simulink model "airTrackLab"  (R2021a)
settings: Solver=ode23t  StartTime=0.0  StopTime=30  FixedStep=0.02  MaxStep=0.01  RelTol=1e-3  AbsTol=1e-4  EnableMultiTasking=on
PostLoadFcn:
  | disp('default settings')
  | 
  | % Default starting positions
  | x0_cart1 = -0.2
  | x0_cart2 = 0.8
  | x0_gate1 = -0.4
  | x0_gate2 = 0.4
  | 
  | % How much damping the carts feel
  | dampingCoef = 0.01 % N/(m/s)
  | 
  | % Hanger damping
  | pulleyDamping = 0;
  | 
  | % Max measurement noise for the gates
  | noise_max = 0.01 % seconds
  | 
  | % How many time steps to show in the history
  | nHistory = 4
  | 
  | % Based on the provided STLs
  | cart_length = 0.15
  | 
  | subsystems = find_system(gcs,'BlockType','SubSystem');
  | p = Simulink.Mask.get(subsystems{1});
  | p.Parameters(1).Value = '-0.8';
  | p.Parameters(2).Value = '0';
  | p.Parameters(3).Value = '-0.4';
  | p.Parameters(4).Value = '0.4';
  | p.Parameters(5).Value = '0';
  | p.Parameters(6).Value = '0';
  | 
  | % Resize the model window
  | set(0,"Units","pixels")
  | sSize = get(0,"screensize");
  | set_param(gcs,'location',...
  |     [1,sSize(4)*0.01,round(sSize(3)/2),sSize(4)*0.96]);
  | 
  | % Reset the zoom
  | set_param(gcs, 'ZoomFactor','FitSystem')
undefined symbols (not defined in the file): X, Y, Z
libraries: sm_lib x104, simulink x12, nesl_utility x9
(part 2 of 3)

== system airTrackLab/Air track model/Endstop R ==
  File Solid2 : sm_lib/Body Elements/File Solid  ExtGeomFileName=wheel_stop.stl  UnitType=Custom  ExtGeomFileUnits=mm  StepReaderType=HEX  ExportConvexHullGeometry=off  InertiaType=PointMass  Mass=180  MassUnits=g  CenterOfMass=[0 0 0]  CenterOfMassUnits=m  MomentsOfInertia=[1 1 1]  MomentsOfInertiaUnits=kg*m^2  ProductsOfInertia=[0 0 0]  ProductsOfInertiaUnits=kg*m^2  BasedOnType=Density  Density=1000  DensityUnits=kg/m^3  DoExposeReferenceFrame=on  SerializedFrames=<Frames><Frame><Id>Frame1</Id><Value><Name>F1</Name><Origin><Source>CenterOfMassFrame</Source><FeatureName></FeatureName></Origin><PrimaryAxis><DefinedDirection>+X</DefinedDirection><Source>ReferenceFrame</Source><SourceDirection>+Z</SourceDirection><FeatureName></FeatureName></PrimaryAxis><SecondaryAxis><DefinedDirection>+Y</DefinedDirection><Source>ReferenceFrame</Source><SourceDirection>+X</SourceDirection><FeatureName></FeatureName></SecondaryAxis></Value></Frame></Frames>  GraphicType=FromGeometry  MarkerShape=Sphere  MarkerSize=10  GraphicVisPropType=AdvancedVisualProperties  GraphicDiffuseColor="[0.2   0.2    0.2]"  GraphicSpecularColor="[0.8    0.8   0.8 1]"  GraphicAmbientColor=[0.05 0.05 0.05 1]  GraphicEmissiveColor=[0.0 0.0 0.0 1.0]  GraphicShininess=50  GraphicOpacity=1.0
  Rigid Transform1 : sm_lib/Frames and Transforms/Rigid Transform  TranslationMethod=Cartesian  TranslationStandardOffset=1  TranslationLengthUnit=m  TranslationStandardAxis=+X  TranslationCartesianOffset=[1-0.012 -0.225 0]  TranslationROffset=0  TranslationROffsetUnits=m  TranslationZOffset=0  TranslationZOffsetUnits=m  TranslationThetaOffset=0  TranslationThetaOffsetUnits=deg  RotationMethod=None  RotationAngleUnits=deg  RotationStandardAxis=+Z  RotationAngle=0.0  RotationArbitraryAxis=[0 0 1]  FollAlignAxisA=+X  BaseAlignAxisA=+Y  FollAlignAxisB=+Y  BaseAlignAxisB=+Z  RotationSequenceAxes=FollowerAxes  RotationSequence=XYX  RotationSequenceAngles=[0 0 0]  RotationSequenceAnglesUnits=deg  RotationMatrix=[1 0 0; 0 1 0; 0 0 1]
  contact_ball1 : sm_lib/Body Elements/Spherical Solid  GraphicAmbientColor=[0.15 0.15 0.15 1.0]  BasedOnType=Density  CenterOfMass=[0 0 0]  CenterOfMassUnits=m  GraphicDiffuseColor="[ 0.9290    0.6940    0.1250]"  Density=1000  DensityUnits=kg/m^3  DoExposeReferenceFrame=on  GraphicEmissiveColor=[0.0 0.0 0.0 1.0]  ExportEntireGeometry=on  SerializedExposedGeometries=<ExposedGeometries><ExposedGeometry><RawGeometryId>entire</RawGeometryId><ExposedGeometryId>G</ExposedGeometryId></ExposedGeometry></ExposedGeometries>  SerializedFrames=<Frames/>  MarkerShape=Sphere  MarkerSize=10  GraphicType=FromGeometry  InertiaType=CalculateFromGeometry  Mass=1  MassUnits=kg  MomentsOfInertia=[1 1 1]  MomentsOfInertiaUnits=kg*m^2  GraphicOpacity=1.0  ProductsOfInertia=[0 0 0]  ProductsOfInertiaUnits=kg*m^2  GraphicShininess=75  GraphicSpecularColor=[0.5 0.5 0.5 1.0]  SphereRadius=0.0075  SphereRadiusUnits=m  GraphicVisPropType=SimpleVisualProperties
  C : PMIOPort  Side=Left
  R : PMIOPort  Port=2  Side=Right
  connections:
  File Solid2/RConn1 -- C/RConn1 -- Rigid Transform1/RConn1 -- R/RConn1
  contact_ball1/RConn1 -- Rigid Transform1/LConn1

== system airTrackLab/Air track model/Force Cart 1 ==
  Add1 : Sum  Inputs=+++
  Force Factor : Gain  Gain=0.5
  Push+ : Constant  SampleTime=-1
  Push- : Constant  Value=-1  SampleTime=-1
  Simulink-PS Converter : nesl_utility/Simulink-PS Converter  PhysicalDomain=network_engine_domain  SubClassName=ps_input  LeftPortType=input  RightPortType=output  PseudoPeriodic=off  Frequencies=[]  NoiseDistribution=none  NoiseParameters=[]  Unit=1  AffineConversion=off  FilteringAndDerivatives=provide  SimscapeFilterOrder=1  InputFilterTimeConstant=0.001  UdotUserProvided=0
      settings: SourceProductBaseCode=PW,SS
  on1+ : Gain  Gain=0
  on1- : Gain  Gain=0
  short pulse : Subsystem
  f : PMIOPort  Side=Right
  wires:
  Force Factor/1 -> Simulink-PS Converter/1
  on1+/1 -> Add1/2
  Push-/1 -> on1-/1
  Push+/1 -> on1+/1
  on1-/1 -> Add1/1
  Add1/1 -> Force Factor/1
  short pulse/1(Out1) -> Add1/3
  connections:
  Simulink-PS Converter/RConn1 -- f/RConn1

== system airTrackLab/Air track model/Force Cart 2 ==
  Add : Sum  Inputs=+++
  Force Factor C2 : Gain  Gain=0.5
  Interactive Pulse : Subsystem
  Push+ : Constant  SampleTime=-1
  Push- : Constant  Value=-1  SampleTime=-1
  Simulink-PS Converter1 : nesl_utility/Simulink-PS Converter  PhysicalDomain=network_engine_domain  SubClassName=ps_input  LeftPortType=input  RightPortType=output  PseudoPeriodic=off  Frequencies=[]  NoiseDistribution=none  NoiseParameters=[]  Unit=1  AffineConversion=off  FilteringAndDerivatives=provide  SimscapeFilterOrder=1  InputFilterTimeConstant=0.001  UdotUserProvided=0
      settings: SourceProductBaseCode=PW,SS
  on2+ : Gain  Gain=0
  on2- : Gain  Gain=0
  f : PMIOPort  Side=Right
  wires:
  Add/1 -> Force Factor C2/1
  Interactive Pulse/1(Out1) -> Add/3
  Force Factor C2/1 -> Simulink-PS Converter1/1
  Push+/1 -> on2+/1
  Push-/1 -> on2-/1
  on2-/1 -> Add/1
  on2+/1 -> Add/2
  connections:
  f/RConn1 -- Simulink-PS Converter1/RConn1

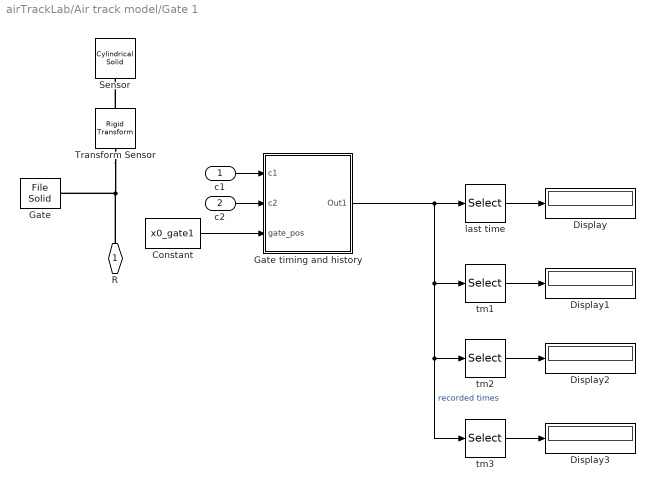
== system airTrackLab/Air track model/Gate 1 ==
  c1 : Inport
  c2 : Inport  Port=2
  Constant : Constant  Value=x0_gate1
  Display{,1..3} (4 alike) : Display
  Gate : sm_lib/Body Elements/File Solid  ExtGeomFileName=gate.stl  UnitType=Custom  ExtGeomFileUnits=mm  StepReaderType=HEX  ExportConvexHullGeometry=off  InertiaType=PointMass  Mass=180  MassUnits=g  CenterOfMass=[0 0 0]  CenterOfMassUnits=m  MomentsOfInertia=[1 1 1]  MomentsOfInertiaUnits=kg*m^2  ProductsOfInertia=[0 0 0]  ProductsOfInertiaUnits=kg*m^2  BasedOnType=Density  Density=1000  DensityUnits=kg/m^3  DoExposeReferenceFrame=on  SerializedFrames=<Frames/>  GraphicType=FromGeometry  MarkerShape=Sphere  MarkerSize=10  GraphicVisPropType=SimpleVisualProperties  GraphicDiffuseColor="[0.8500    0.3250    0.0980]"  GraphicSpecularColor="[0.8    0.8   0.8 1]"  GraphicAmbientColor=[0.05 0.05 0.05 1]  GraphicEmissiveColor=[0.0 0.0 0.0 1.0]  GraphicShininess=50  GraphicOpacity=0.5
  Gate timing and history : Subsystem
  Sensor : sm_lib/Body Elements/Cylindrical Solid  GraphicAmbientColor=[0.15 0.15 0.15 1.0]  BasedOnType=Density  CenterOfMass=[0 0 0]  CenterOfMassUnits=m  GraphicDiffuseColor=[0.0 0.6 0.0]  CylinderLength=0.008  CylinderLengthUnits=m  CylinderRadius=0.01  CylinderRadiusUnits=m  Density=1000  DensityUnits=kg/m^3  DoExposeReferenceFrame=on  GraphicEmissiveColor=[0.0 0.0 0.0 1.0]  ExportEntireGeometry=off  SerializedFrames=<Frames/>  MarkerShape=Sphere  MarkerSize=10  GraphicType=FromGeometry  InertiaType=CalculateFromGeometry  Mass=1  MassUnits=kg  MomentsOfInertia=[1 1 1]  MomentsOfInertiaUnits=kg*m^2  GraphicOpacity=1.0  ProductsOfInertia=[0 0 0]  ProductsOfInertiaUnits=kg*m^2  GraphicShininess=75  GraphicSpecularColor=[0.5 0.5 0.5 1.0]  GraphicVisPropType=SimpleVisualProperties
  Transform Sensor : sm_lib/Frames and Transforms/Rigid Transform  TranslationMethod=StandardAxis  TranslationStandardOffset=0.2675  TranslationLengthUnit=m  TranslationStandardAxis=+Y  TranslationCartesianOffset=[0 0 0]  TranslationROffset=0  TranslationROffsetUnits=m  TranslationZOffset=0  TranslationZOffsetUnits=m  TranslationThetaOffset=0  TranslationThetaOffsetUnits=deg  RotationMethod=StandardAxis  RotationAngleUnits=deg  RotationStandardAxis=+X  RotationAngle=-90  RotationArbitraryAxis=[0 0 1]  FollAlignAxisA=+X  BaseAlignAxisA=+Y  FollAlignAxisB=+Y  BaseAlignAxisB=+Z  RotationSequenceAxes=FollowerAxes  RotationSequence=XYX  RotationSequenceAngles=[0 0 0]  RotationSequenceAnglesUnits=deg  RotationMatrix=[1 0 0; 0 1 0; 0 0 1]
  last time : Selector  InputPortWidth=4  IndexOptions=Index vector (dialog)  Indices=1  OutputSizes=1
  tm1 : Selector  InputPortWidth=4  IndexOptions=Index vector (dialog)  Indices=2  OutputSizes=1
  tm2 : Selector  InputPortWidth=4  IndexOptions=Index vector (dialog)  Indices=3  OutputSizes=1
  tm3 : Selector  InputPortWidth=4  IndexOptions=Index vector (dialog)  Indices=4  OutputSizes=1
  R : PMIOPort  Side=Right
  wires:
  Gate timing and history/1(Out1) -> tm3/1, tm2/1, tm1/1, last time/1  "recorded times"
  Constant/1 -> Gate timing and history/3(gate_pos)
  c1/1 -> Gate timing and history/1(c1)
  c2/1 -> Gate timing and history/2(c2)
  last time/1 -> Display/1
  tm1/1 -> Display1/1
  tm2/1 -> Display2/1
  tm3/1 -> Display3/1
  connections:
  R/RConn1 -- Transform Sensor/LConn1 -- Gate/RConn1
  Transform Sensor/RConn1 -- Sensor/RConn1

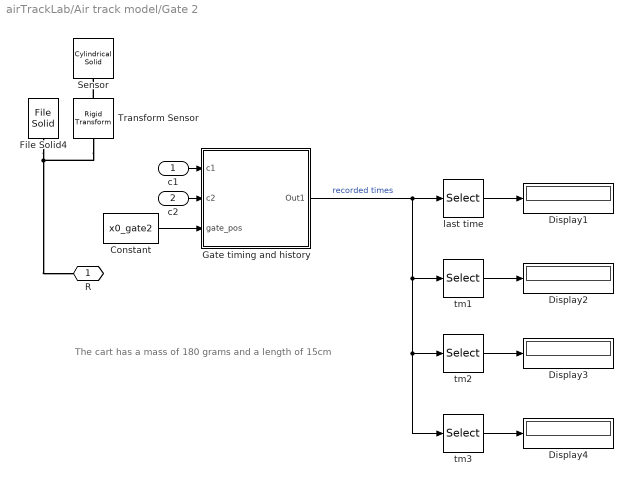
== system airTrackLab/Air track model/Gate 2 ==
  note: The cart has a mass of 180 grams and a length of 15cm
  c1 : Inport
  c2 : Inport  Port=2
  Constant : Constant  Value=x0_gate2
  Display{1..4} (4 alike) : Display
  File Solid4 : sm_lib/Body Elements/File Solid  ExtGeomFileName=gate.stl  UnitType=Custom  ExtGeomFileUnits=mm  StepReaderType=HEX  ExportConvexHullGeometry=off  InertiaType=PointMass  Mass=180  MassUnits=g  CenterOfMass=[0 0 0]  CenterOfMassUnits=m  MomentsOfInertia=[1 1 1]  MomentsOfInertiaUnits=kg*m^2  ProductsOfInertia=[0 0 0]  ProductsOfInertiaUnits=kg*m^2  BasedOnType=Density  Density=1000  DensityUnits=kg/m^3  DoExposeReferenceFrame=on  SerializedFrames=<Frames/>  GraphicType=FromGeometry  MarkerShape=Sphere  MarkerSize=10  GraphicVisPropType=SimpleVisualProperties  GraphicDiffuseColor="[           0    0.4470    0.7410]"  GraphicSpecularColor="[0.8    0.8   0.8 1]"  GraphicAmbientColor=[0.05 0.05 0.05 1]  GraphicEmissiveColor=[0.0 0.0 0.0 1.0]  GraphicShininess=50  GraphicOpacity=0.5
  Gate timing and history : Subsystem
  Sensor : sm_lib/Body Elements/Cylindrical Solid  GraphicAmbientColor=[0.15 0.15 0.15 1.0]  BasedOnType=Density  CenterOfMass=[0 0 0]  CenterOfMassUnits=m  GraphicDiffuseColor=[0.0 0.6 0.0]  CylinderLength=0.008  CylinderLengthUnits=m  CylinderRadius=0.01  CylinderRadiusUnits=m  Density=1000  DensityUnits=kg/m^3  DoExposeReferenceFrame=on  GraphicEmissiveColor=[0.0 0.0 0.0 1.0]  ExportEntireGeometry=off  SerializedFrames=<Frames/>  MarkerShape=Sphere  MarkerSize=10  GraphicType=FromGeometry  InertiaType=CalculateFromGeometry  Mass=1  MassUnits=kg  MomentsOfInertia=[1 1 1]  MomentsOfInertiaUnits=kg*m^2  GraphicOpacity=1.0  ProductsOfInertia=[0 0 0]  ProductsOfInertiaUnits=kg*m^2  GraphicShininess=75  GraphicSpecularColor=[0.5 0.5 0.5 1.0]  GraphicVisPropType=SimpleVisualProperties
  Transform Sensor : sm_lib/Frames and Transforms/Rigid Transform  TranslationMethod=StandardAxis  TranslationStandardOffset=0.2675  TranslationLengthUnit=m  TranslationStandardAxis=+Y  TranslationCartesianOffset=[0 0 0]  TranslationROffset=0  TranslationROffsetUnits=m  TranslationZOffset=0  TranslationZOffsetUnits=m  TranslationThetaOffset=0  TranslationThetaOffsetUnits=deg  RotationMethod=StandardAxis  RotationAngleUnits=deg  RotationStandardAxis=+X  RotationAngle=-90  RotationArbitraryAxis=[0 0 1]  FollAlignAxisA=+X  BaseAlignAxisA=+Y  FollAlignAxisB=+Y  BaseAlignAxisB=+Z  RotationSequenceAxes=FollowerAxes  RotationSequence=XYX  RotationSequenceAngles=[0 0 0]  RotationSequenceAnglesUnits=deg  RotationMatrix=[1 0 0; 0 1 0; 0 0 1]
  last time : Selector  InputPortWidth=4  IndexOptions=Index vector (dialog)  Indices=1  OutputSizes=1
  tm1 : Selector  InputPortWidth=4  IndexOptions=Index vector (dialog)  Indices=2  OutputSizes=1
  tm2 : Selector  InputPortWidth=4  IndexOptions=Index vector (dialog)  Indices=3  OutputSizes=1
  tm3 : Selector  InputPortWidth=4  IndexOptions=Index vector (dialog)  Indices=4  OutputSizes=1
  R : PMIOPort  Side=Right
  wires:
  Constant/1 -> Gate timing and history/3(gate_pos)
  c1/1 -> Gate timing and history/1(c1)
  c2/1 -> Gate timing and history/2(c2)
  Gate timing and history/1(Out1) -> tm3/1, tm2/1, tm1/1, last time/1  "recorded times"
  tm1/1 -> Display2/1
  tm3/1 -> Display4/1
  last time/1 -> Display1/1
  tm2/1 -> Display3/1
  connections:
  File Solid4/RConn1 -- Transform Sensor/LConn1 -- R/RConn1
  Transform Sensor/RConn1 -- Sensor/RConn1

== system airTrackLab/Air track model/Load ==
  Hanging Mass : Subsystem  VariantControl=Hanging_Mass
  None : Subsystem  VariantControl=None
  Cable : PMIOPort  Side=Left
  Bracket : PMIOPort  Port=2  Side=Left

== system airTrackLab/Air track model/Mass Cart 1 ==
  "None " : Subsystem  VariantControl=None
      mask Display: disp(' ');
  Plates 1 : Subsystem  VariantControl=Plates_1
      mask Display: image('Plates_1.png');
  Plates 2 : Subsystem  VariantControl=Plates_2
      mask Display: image('Plates_2.png');
  Plates 3 : Subsystem  VariantControl=Plates_3
      mask Display: image('Plates_3.png');
  B : PMIOPort  Side=Right

== system airTrackLab/Air track model/Mass Cart 2 ==
  "None " : Subsystem  VariantControl=None
      mask Display: disp(' ');
  Plates 1 : Subsystem  VariantControl=Plates_1
      mask Display: image('Plates_1.png');
  Plates 2 : Subsystem  VariantControl=Plates_2
      mask Display: image('Plates_2.png');
  Plates 3 : Subsystem  VariantControl=Plates_3
      mask Display: image('Plates_3.png');
  B : PMIOPort  Side=Right

== system airTrackLab/Air track model/Subsystem1 ==
  Bus Creator : BusCreator  Inputs=2
  PS-Simulink Converter : nesl_utility/PS-Simulink Converter  PhysicalDomain=network_engine_domain  SubClassName=ps_output  LeftPortType=input  RightPortType=output  PseudoPeriodic=off  Frequencies=[]  Unit=inherit  AffineConversion=off
      settings: SourceProductBaseCode=PW,SS
  PS-Simulink Converter1 : nesl_utility/PS-Simulink Converter  PhysicalDomain=network_engine_domain  SubClassName=ps_output  LeftPortType=input  RightPortType=output  PseudoPeriodic=off  Frequencies=[]  Unit=inherit  AffineConversion=off
      settings: SourceProductBaseCode=PW,SS
  p : PMIOPort  Side=Left
  v : PMIOPort  Port=2  Side=Left
  pv : Outport
  wires:
  PS-Simulink Converter1/1 -> Bus Creator/1  "p"
  PS-Simulink Converter/1 -> Bus Creator/2  "v"
  Bus Creator/1 -> pv/1  "cart1"
  connections:
  v/RConn1 -- PS-Simulink Converter/LConn1
  p/RConn1 -- PS-Simulink Converter1/LConn1

== system airTrackLab/Air track model/Subsystem4 ==
  Bus Creator : BusCreator  Inputs=2
  PS-Simulink Converter : nesl_utility/PS-Simulink Converter  PhysicalDomain=network_engine_domain  SubClassName=ps_output  LeftPortType=input  RightPortType=output  PseudoPeriodic=off  Frequencies=[]  Unit=inherit  AffineConversion=off
      settings: SourceProductBaseCode=PW,SS
  PS-Simulink Converter1 : nesl_utility/PS-Simulink Converter  PhysicalDomain=network_engine_domain  SubClassName=ps_output  LeftPortType=input  RightPortType=output  PseudoPeriodic=off  Frequencies=[]  Unit=inherit  AffineConversion=off
      settings: SourceProductBaseCode=PW,SS
  p : PMIOPort  Side=Left
  v : PMIOPort  Port=2  Side=Left
  pv : Outport
  wires:
  Bus Creator/1 -> pv/1  "cart2"
  PS-Simulink Converter/1 -> Bus Creator/2  "v"
  PS-Simulink Converter1/1 -> Bus Creator/1  "p"
  connections:
  PS-Simulink Converter/LConn1 -- v/RConn1
  PS-Simulink Converter1/LConn1 -- p/RConn1

== system airTrackLab/Air track model/Contact Force/Elastic ==
  Contact Force Carts : sm_lib/Forces and Torques/Spatial Contact Force  CoefficientOfDynamicFriction=0.3  CoefficientOfStaticFriction=0.5  SenseContactBaseRotation=off  SenseContactBaseTranslation=off  NormalDamping=1e-3  NormalDampingUnits=N/(m/s)  SenseContactFollowerRotation=off  SenseContactFollowerTranslation=off  SenseContactSignal=off  NormalStiffness=1e9  NormalStiffnessUnits=N/m  FrictionalCriticalVelocity=1e-3  FrictionalCriticalVelocityUnits=m/s  ZeroCrossDetectContactStartAndEnd=off  FrictionType=None  SenseFrictionalForceMagnitude=off  SenseNormalForceMagnitude=off  NormalForceType=SmoothSpringDamper  SenseNormalVelocity=off  SenseSeparationDistance=off  SenseTangentialVelocity=off  SenseTangentialVelocityMagnitude=off  NormalTransitionRegionWidth=1e-4  NormalTransitionRegionWidthUnits=m
  Contact Force Carts1 : sm_lib/Forces and Torques/Spatial Contact Force  CoefficientOfDynamicFriction=0.3  CoefficientOfStaticFriction=0.5  SenseContactBaseRotation=off  SenseContactBaseTranslation=off  NormalDamping=1e-3  NormalDampingUnits=N/(m/s)  SenseContactFollowerRotation=off  SenseContactFollowerTranslation=off  SenseContactSignal=off  NormalStiffness=1e9  NormalStiffnessUnits=N/m  FrictionalCriticalVelocity=1e-3  FrictionalCriticalVelocityUnits=m/s  ZeroCrossDetectContactStartAndEnd=off  FrictionType=None  SenseFrictionalForceMagnitude=off  SenseNormalForceMagnitude=off  NormalForceType=SmoothSpringDamper  SenseNormalVelocity=off  SenseSeparationDistance=off  SenseTangentialVelocity=off  SenseTangentialVelocityMagnitude=off  NormalTransitionRegionWidth=1e-4  NormalTransitionRegionWidthUnits=m
  Reference Frame : sm_lib/Frames and Transforms/Reference Frame
  Reference Frame1 : sm_lib/Frames and Transforms/Reference Frame
  Weld Joint : sm_lib/Joints/Weld Joint  JointMode=ProvidedByInput  SenseConstraintForce=off  SenseConstraintForceX=off  SenseConstraintForceY=off  SenseConstraintForceZ=off  SenseConstraintTorque=off  SenseConstraintTorqueX=off  SenseConstraintTorqueY=off  SenseConstraintTorqueZ=off  SenseTotalForce=off  SenseTotalForceX=off  SenseTotalForceY=off  SenseTotalForceZ=off  SenseTotalTorque=off  SenseTotalTorqueX=off  SenseTotalTorqueY=off  SenseTotalTorqueZ=off  CompositeWrenchDir=FollowerOnBase  CompositeWrenchFrame=BaseFrame
  G1 : PMIOPort  Side=Left
  G2 : PMIOPort  Port=2  Side=Right
  F1 : PMIOPort  Port=3  Side=Left
  F2 : PMIOPort  Port=4  Side=Right
  connections:
  F1/RConn1 -- Reference Frame/RConn1
  F2/RConn1 -- Reference Frame1/RConn1
  G1/RConn1 -- Contact Force Carts/RConn1
  G2/RConn1 -- Contact Force Carts/LConn1

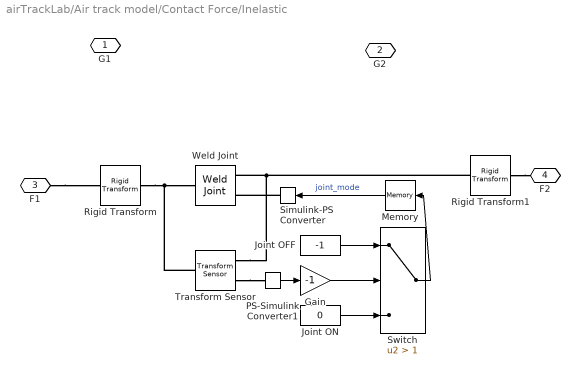
== system airTrackLab/Air track model/Contact Force/Inelastic ==
  Gain : Gain  Gain=-1
  Joint OFF : Constant  Value=-1
  Joint ON : Constant  Value=0
  Memory : Memory  InitialCondition=-1
  PS-Simulink Converter1 : nesl_utility/PS-Simulink Converter  PhysicalDomain=network_engine_domain  SubClassName=ps_output  LeftPortType=input  RightPortType=output  PseudoPeriodic=off  Frequencies=[]  Unit=mm  AffineConversion=off
      settings: SourceProductBaseCode=PW,SS
  Rigid Transform : sm_lib/Frames and Transforms/Rigid Transform  TranslationMethod=StandardAxis  TranslationStandardOffset=-0.075-0.0075  TranslationLengthUnit=m  TranslationStandardAxis=+Z  TranslationCartesianOffset=[0 0 0]  TranslationROffset=0  TranslationROffsetUnits=m  TranslationZOffset=0  TranslationZOffsetUnits=m  TranslationThetaOffset=0  TranslationThetaOffsetUnits=deg  RotationMethod=None  RotationAngleUnits=deg  RotationStandardAxis=+Z  RotationAngle=0.0  RotationArbitraryAxis=[0 0 1]  FollAlignAxisA=+X  BaseAlignAxisA=+Y  FollAlignAxisB=+Y  BaseAlignAxisB=+Z  RotationSequenceAxes=FollowerAxes  RotationSequence=XYX  RotationSequenceAngles=[0 0 0]  RotationSequenceAnglesUnits=deg  RotationMatrix=[1 0 0; 0 1 0; 0 0 1]
  Rigid Transform1 : sm_lib/Frames and Transforms/Rigid Transform  TranslationMethod=StandardAxis  TranslationStandardOffset=0.075+0.0075  TranslationLengthUnit=m  TranslationStandardAxis=+Z  TranslationCartesianOffset=[0 0 0]  TranslationROffset=0  TranslationROffsetUnits=m  TranslationZOffset=0  TranslationZOffsetUnits=m  TranslationThetaOffset=0  TranslationThetaOffsetUnits=deg  RotationMethod=None  RotationAngleUnits=deg  RotationStandardAxis=+Z  RotationAngle=0.0  RotationArbitraryAxis=[0 0 1]  FollAlignAxisA=+X  BaseAlignAxisA=+Y  FollAlignAxisB=+Y  BaseAlignAxisB=+Z  RotationSequenceAxes=FollowerAxes  RotationSequence=XYX  RotationSequenceAngles=[0 0 0]  RotationSequenceAnglesUnits=deg  RotationMatrix=[1 0 0; 0 1 0; 0 0 1]
  Simulink-PS Converter : nesl_utility/Simulink-PS Converter  PhysicalDomain=network_engine_domain  SubClassName=ps_input  LeftPortType=input  RightPortType=output  PseudoPeriodic=off  Frequencies=[]  NoiseDistribution=none  NoiseParameters=[]  Unit=1  AffineConversion=off  FilteringAndDerivatives=provide  SimscapeFilterOrder=1  InputFilterTimeConstant=0.001  UdotUserProvided=0
      settings: SourceProductBaseCode=PW,SS
  Switch : Switch  Criteria=u2 > Threshold  Threshold=1
  Transform Sensor : sm_lib/Frames and Transforms/Transform Sensor  MeasurementFrame=Base  SenseAngle=off  SenseAxis=off  SenseAngle1=off  SenseAngle2=off  SenseAngle3=off  SenseQ=off  SenseR=off  SenseOmegaX=off  SenseOmegaY=off  SenseOmegaZ=off  SenseOmega1=off  SenseOmega2=off  SenseOmega3=off  SenseQDot=off  SenseRDot=off  SenseAlphaX=off  SenseAlphaY=off  SenseAlphaZ=off  SenseAlpha1=off  SenseAlpha2=off  SenseAlpha3=off  SenseQDDot=off  SenseRDDot=off  SenseX=off  SenseY=off  SenseZ=on  SenseRad=off  SenseAzim=off  SenseDist=off  SenseInc=off  SenseXDot=off  SenseYDot=off  SenseZDot=off  SenseRadDot=off  SenseAzimDot=off  SenseDistDot=off  SenseIncDot=off  SenseXDDot=off  SenseYDDot=off  SenseZDDot=off  SenseRadDDot=off  SenseAzimDDot=off  SenseDistDDot=off  SenseIncDDot=off
  Weld Joint : sm_lib/Joints/Weld Joint  JointMode=ProvidedByInput  SenseConstraintForce=off  SenseConstraintForceX=off  SenseConstraintForceY=off  SenseConstraintForceZ=off  SenseConstraintTorque=off  SenseConstraintTorqueX=off  SenseConstraintTorqueY=off  SenseConstraintTorqueZ=off  SenseTotalForce=off  SenseTotalForceX=off  SenseTotalForceY=off  SenseTotalForceZ=off  SenseTotalTorque=off  SenseTotalTorqueX=off  SenseTotalTorqueY=off  SenseTotalTorqueZ=off  CompositeWrenchDir=FollowerOnBase  CompositeWrenchFrame=BaseFrame
  G1 : PMIOPort  Side=Left
  G2 : PMIOPort  Port=2  Side=Right
  F1 : PMIOPort  Port=3  Side=Left
  F2 : PMIOPort  Port=4  Side=Right
  wires:
  Joint OFF/1 -> Switch/1
  Joint ON/1 -> Switch/3
  Memory/1 -> Simulink-PS Converter/1  "joint_mode"
  Switch/1 -> Memory/1
  PS-Simulink Converter1/1 -> Gain/1
  Gain/1 -> Switch/2
  connections:
  Rigid Transform1/LConn1 -- F2/RConn1
  Simulink-PS Converter/RConn1 -- Weld Joint/LConn2
  F1/RConn1 -- Rigid Transform/LConn1
  Rigid Transform/RConn1 -- Transform Sensor/LConn1 -- Weld Joint/RConn1
  Rigid Transform1/RConn1 -- Transform Sensor/RConn1 -- Weld Joint/LConn1
  Transform Sensor/RConn2 -- PS-Simulink Converter1/LConn1

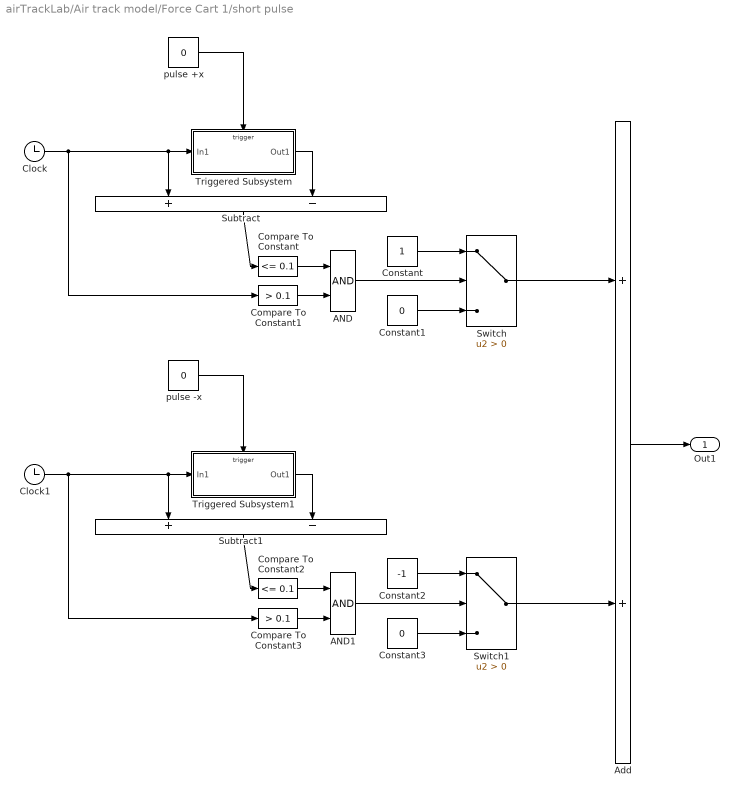
== system airTrackLab/Air track model/Force Cart 1/short pulse ==
  AND : Logic  IconShape=distinctive  AllPortsSameDT=off  OutDataTypeStr=boolean
  AND1 : Logic  IconShape=distinctive  AllPortsSameDT=off  OutDataTypeStr=boolean
  Add : Sum
  Clock : Clock
  Clock1 : Clock
  Compare To Constant : simulink/Logic and Bit Operations/Compare To Constant  relop=<=  const=0.1  OutDataTypeStr=boolean
  Compare To Constant1 : simulink/Logic and Bit Operations/Compare To Constant  relop=>  const=0.1  OutDataTypeStr=boolean
  Compare To Constant2 : simulink/Logic and Bit Operations/Compare To Constant  relop=<=  const=0.1  OutDataTypeStr=boolean
  Compare To Constant3 : simulink/Logic and Bit Operations/Compare To Constant  relop=>  const=0.1  OutDataTypeStr=boolean
  Constant : Constant
  Constant1 : Constant  Value=0
  Constant2 : Constant  Value=-1
  Constant3 : Constant  Value=0
  Subtract : Sum  Inputs=+-
  Subtract1 : Sum  Inputs=+-
  Switch : Switch  Criteria=u2 > Threshold
  Switch1 : Switch  Criteria=u2 > Threshold
  Triggered Subsystem : Subsystem  TreatAsAtomicUnit=on
  Triggered Subsystem1 : Subsystem  TreatAsAtomicUnit=on
  pulse +x : Constant  Value=0
  pulse -x : Constant  Value=0
  Out1 : Outport
  wires:
  pulse +x/1 -> Triggered Subsystem/Trigger
  Triggered Subsystem/1(Out1) -> Subtract/2
  Constant/1 -> Switch/1
  Subtract/1 -> Compare To Constant/1
  Constant1/1 -> Switch/3
  AND/1 -> Switch/2
  Compare To Constant/1 -> AND/1
  Clock/1 -> Compare To Constant1/1, Triggered Subsystem/1(In1), Subtract/1
  Compare To Constant1/1 -> AND/2
  Switch/1 -> Add/1
  Add/1 -> Out1/1
  Compare To Constant3/1 -> AND1/2
  Switch1/1 -> Add/2
  pulse -x/1 -> Triggered Subsystem1/Trigger
  Clock1/1 -> Compare To Constant3/1, Triggered Subsystem1/1(In1), Subtract1/1
  Constant3/1 -> Switch1/3
  Compare To Constant2/1 -> AND1/1
  Subtract1/1 -> Compare To Constant2/1
  Constant2/1 -> Switch1/1
  AND1/1 -> Switch1/2
  Triggered Subsystem1/1(Out1) -> Subtract1/2

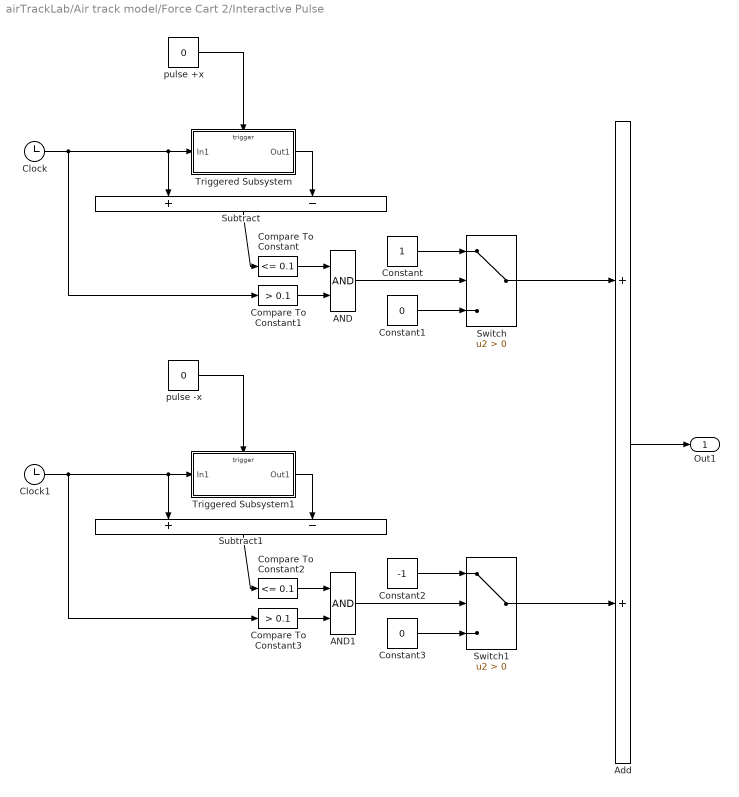
== system airTrackLab/Air track model/Force Cart 2/Interactive Pulse ==
  AND : Logic  IconShape=distinctive  AllPortsSameDT=off  OutDataTypeStr=boolean
  AND1 : Logic  IconShape=distinctive  AllPortsSameDT=off  OutDataTypeStr=boolean
  Add : Sum
  Clock : Clock
  Clock1 : Clock
  Compare To Constant : simulink/Logic and Bit Operations/Compare To Constant  relop=<=  const=0.1  OutDataTypeStr=boolean
  Compare To Constant1 : simulink/Logic and Bit Operations/Compare To Constant  relop=>  const=0.1  OutDataTypeStr=boolean
  Compare To Constant2 : simulink/Logic and Bit Operations/Compare To Constant  relop=<=  const=0.1  OutDataTypeStr=boolean
  Compare To Constant3 : simulink/Logic and Bit Operations/Compare To Constant  relop=>  const=0.1  OutDataTypeStr=boolean
  Constant : Constant
  Constant1 : Constant  Value=0
  Constant2 : Constant  Value=-1
  Constant3 : Constant  Value=0
  Subtract : Sum  Inputs=+-
  Subtract1 : Sum  Inputs=+-
  Switch : Switch  Criteria=u2 > Threshold
  Switch1 : Switch  Criteria=u2 > Threshold
  Triggered Subsystem : Subsystem  TreatAsAtomicUnit=on
  Triggered Subsystem1 : Subsystem  TreatAsAtomicUnit=on
  pulse +x : Constant  Value=0
  pulse -x : Constant  Value=0
  Out1 : Outport
  wires:
  pulse +x/1 -> Triggered Subsystem/Trigger
  Triggered Subsystem/1(Out1) -> Subtract/2
  Constant/1 -> Switch/1
  Subtract/1 -> Compare To Constant/1
  Constant1/1 -> Switch/3
  AND/1 -> Switch/2
  Compare To Constant/1 -> AND/1
  Clock/1 -> Compare To Constant1/1, Triggered Subsystem/1(In1), Subtract/1
  Compare To Constant1/1 -> AND/2
  Switch/1 -> Add/1
  Add/1 -> Out1/1
  Compare To Constant3/1 -> AND1/2
  Switch1/1 -> Add/2
  pulse -x/1 -> Triggered Subsystem1/Trigger
  Clock1/1 -> Compare To Constant3/1, Triggered Subsystem1/1(In1), Subtract1/1
  Constant3/1 -> Switch1/3
  Compare To Constant2/1 -> AND1/1
  Subtract1/1 -> Compare To Constant2/1
  Constant2/1 -> Switch1/1
  AND1/1 -> Switch1/2
  Triggered Subsystem1/1(Out1) -> Subtract1/2

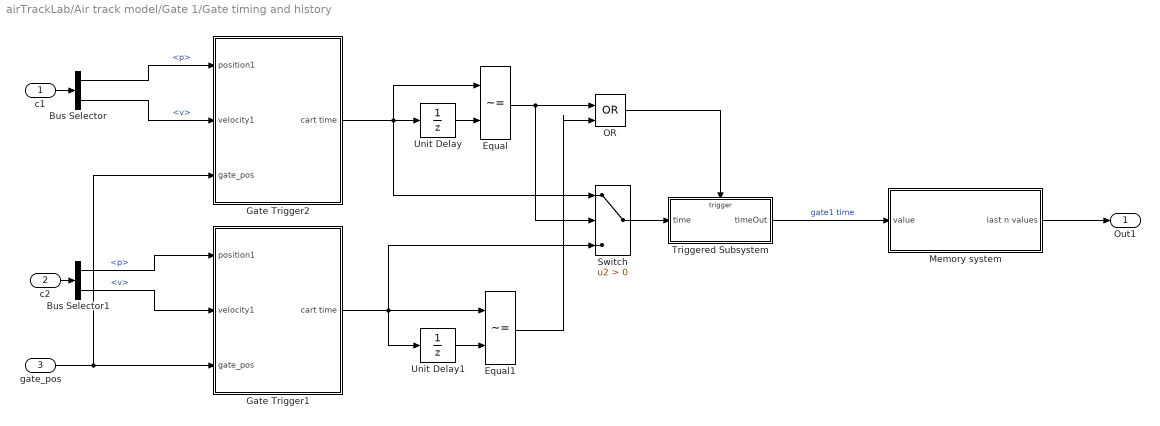
== system airTrackLab/Air track model/Gate 1/Gate timing and history ==
  c1 : Inport
  c2 : Inport  Port=2
  gate_pos : Inport  Port=3
  Bus Selector : BusSelector  OutputSignals=p,v
  Bus Selector1 : BusSelector  OutputSignals=p,v
  Equal : RelationalOperator  Operator=~=  OutDataTypeStr=boolean  RndMeth=Simplest
  Equal1 : RelationalOperator  Operator=~=  OutDataTypeStr=boolean  RndMeth=Simplest
  Gate Trigger1 : Subsystem
  Gate Trigger2 : Subsystem
  Memory system : Subsystem
  OR : Logic  Operator=OR  IconShape=distinctive  AllPortsSameDT=off  OutDataTypeStr=boolean
  Switch : Switch  Criteria=u2 > Threshold
  Triggered Subsystem : Subsystem  TreatAsAtomicUnit=on
  Unit Delay : UnitDelay  SampleTime=-1  HasFrameUpgradeWarning=on
  Unit Delay1 : UnitDelay  SampleTime=-1  HasFrameUpgradeWarning=on
  Out1 : Outport
  wires:
  Gate Trigger1/1(cart time) -> Switch/3, Equal1/1, Unit Delay1/1
  gate_pos/1 -> Gate Trigger2/3(gate_pos), Gate Trigger1/3(gate_pos)
  OR/1 -> Triggered Subsystem/Trigger
  Bus Selector1/1 -> Gate Trigger1/1(position1)  "<p>"
  Equal/1 -> Switch/2, OR/1
  Triggered Subsystem/1(timeOut) -> Memory system/1(value)  "gate1 time"
  Bus Selector1/2 -> Gate Trigger1/2(velocity1)  "<v>"
  Unit Delay/1 -> Equal/2
  Gate Trigger2/1(cart time) -> Switch/1, Equal/1, Unit Delay/1
  Equal1/1 -> OR/2
  Unit Delay1/1 -> Equal1/2
  Bus Selector/1 -> Gate Trigger2/1(position1)  "<p>"
  Switch/1 -> Triggered Subsystem/1(time)
  Memory system/1(last n values) -> Out1/1
  c1/1 -> Bus Selector/1
  Bus Selector/2 -> Gate Trigger2/2(velocity1)  "<v>"
  c2/1 -> Bus Selector1/1

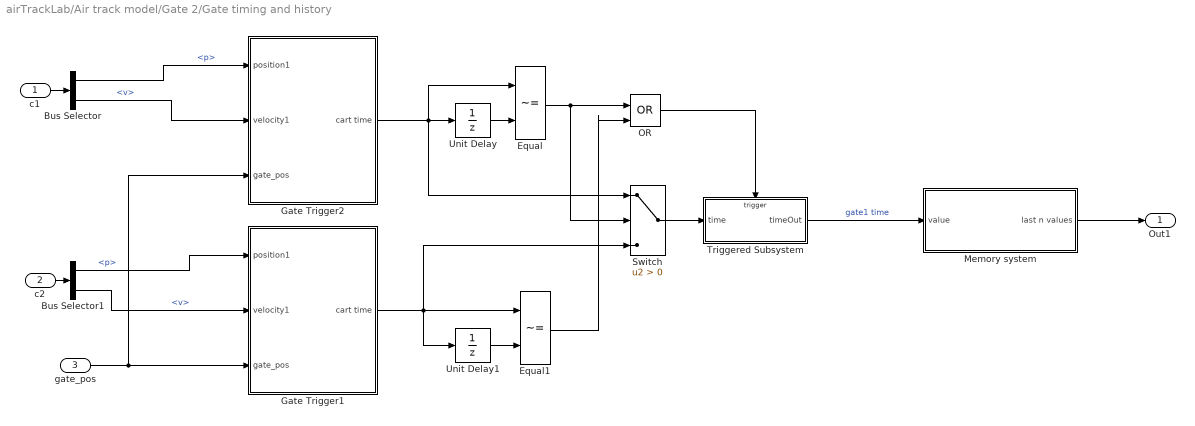
== system airTrackLab/Air track model/Gate 2/Gate timing and history ==
  c1 : Inport
  c2 : Inport  Port=2
  gate_pos : Inport  Port=3
  Bus Selector : BusSelector  OutputSignals=p,v
  Bus Selector1 : BusSelector  OutputSignals=p,v
  Equal : RelationalOperator  Operator=~=  OutDataTypeStr=boolean  RndMeth=Simplest
  Equal1 : RelationalOperator  Operator=~=  OutDataTypeStr=boolean  RndMeth=Simplest
  Gate Trigger1 : Subsystem
  Gate Trigger2 : Subsystem
  Memory system : Subsystem
  OR : Logic  Operator=OR  IconShape=distinctive  AllPortsSameDT=off  OutDataTypeStr=boolean
  Switch : Switch  Criteria=u2 > Threshold
  Triggered Subsystem : Subsystem  TreatAsAtomicUnit=on
  Unit Delay : UnitDelay  SampleTime=-1  HasFrameUpgradeWarning=on
  Unit Delay1 : UnitDelay  SampleTime=-1  HasFrameUpgradeWarning=on
  Out1 : Outport
  wires:
  Gate Trigger1/1(cart time) -> Switch/3, Equal1/1, Unit Delay1/1
  gate_pos/1 -> Gate Trigger2/3(gate_pos), Gate Trigger1/3(gate_pos)
  OR/1 -> Triggered Subsystem/Trigger
  Equal/1 -> Switch/2, OR/1
  Triggered Subsystem/1(timeOut) -> Memory system/1(value)  "gate1 time"
  Unit Delay/1 -> Equal/2
  Gate Trigger2/1(cart time) -> Switch/1, Equal/1, Unit Delay/1
  Equal1/1 -> OR/2
  Unit Delay1/1 -> Equal1/2
  Switch/1 -> Triggered Subsystem/1(time)
  Memory system/1(last n values) -> Out1/1
  Bus Selector/1 -> Gate Trigger2/1(position1)  "<p>"
  Bus Selector/2 -> Gate Trigger2/2(velocity1)  "<v>"
  c1/1 -> Bus Selector/1
  Bus Selector1/1 -> Gate Trigger1/1(position1)  "<p>"
  Bus Selector1/2 -> Gate Trigger1/2(velocity1)  "<v>"
  c2/1 -> Bus Selector1/1

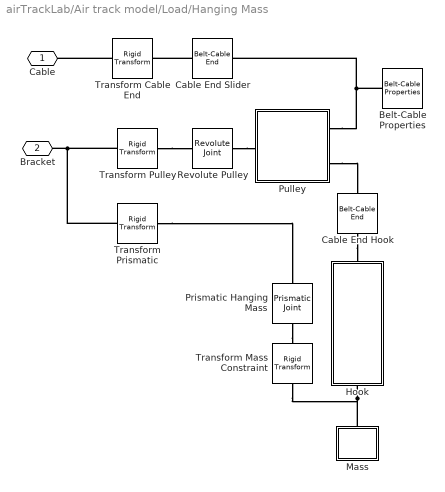
== system airTrackLab/Air track model/Load/Hanging Mass ==
  Belt-Cable Properties : sm_lib/Belts and Cables/Belt-Cable Properties  DrumBeltCableAlignment=MonitoredPlanar  GraphicType=PitchLine  GraphicVisPropType=SimpleVisualProperties  GraphicDiffuseColor=[1.0 0.0 0.0]  GraphicSpecularColor=[0.5 0.5 0.5 1.0]  GraphicAmbientColor=[0.15 0.15 0.15 1.0]  GraphicEmissiveColor=[0.0 0.0 0.0 1.0]  GraphicShininess=75  GraphicOpacity=1.0
      settings: SourceProductBaseCode=MS
  Cable End Hook : sm_lib/Belts and Cables/Belt-Cable End
      settings: SourceProductBaseCode=MS
  Cable End Slider : sm_lib/Belts and Cables/Belt-Cable End
      settings: SourceProductBaseCode=MS
  Hook : Subsystem
      mask Display: image('hangingMassHook.png');
  Mass : Subsystem  Variant=on  VariantControlMode=label  VariantControl=Choice  LabelModeActiveChoice=Plates_1
      settings: AttributesFormatString=%<LabelModeActiveChoice>
  Prismatic Hanging Mass : sm_lib/Joints/Prismatic Joint  JointMode=Normal  SenseConstraintForce=off  SenseConstraintForceX=off  SenseConstraintForceY=off  SenseConstraintForceZ=off  SenseConstraintTorque=off  SenseConstraintTorqueX=off  SenseConstraintTorqueY=off  SenseConstraintTorqueZ=off  SenseTotalForce=off  SenseTotalForceX=off  SenseTotalForceY=off  SenseTotalForceZ=off  SenseTotalTorque=off  SenseTotalTorqueX=off  SenseTotalTorqueY=off  SenseTotalTorqueZ=off  CompositeWrenchDir=FollowerOnBase  CompositeWrenchFrame=BaseFrame  EquilibriumPosition=0  EquilibriumPositionUnits=m  SpringStiffness=0  SpringStiffnessUnits=N/m  DampingCoefficient=0  DampingCoefficientUnits=N/(m/s)  TorqueActuationMode=NoTorque  MotionActuationMode=ComputedMotion  SensePosition=off  SenseVelocity=off  SenseAcceleration=off  SenseTorqueForce=off  SenseLowerLimitTorqueForce=off  SenseUpperLimitTorqueForce=off  LowerLimitSpecify=off  LowerLimitBound=-1  LowerLimitBoundUnits=m  LowerLimitStiffness=1e6  LowerLimitStiffnessUnits=N/m  LowerLimitDamping=1e3  LowerLimitDampingUnits=N/(m/s)  LowerLimitTransitionRegionWidth=1e-4  LowerLimitTransitionRegionWidthUnits=m  UpperLimitSpecify=off  UpperLimitBound=1  UpperLimitBoundUnits=m  UpperLimitStiffness=1e6  UpperLimitStiffnessUnits=N/m  UpperLimitDamping=1e3  UpperLimitDampingUnits=N/(m/s)  UpperLimitTransitionRegionWidth=1e-4  UpperLimitTransitionRegionWidthUnits=m  PositionTargetSpecify=off  PositionTargetPriority=High  PositionTargetValue=0  PositionTargetValueUnits=m  VelocityTargetSpecify=off  VelocityTargetPriority=High  VelocityTargetValue=0  VelocityTargetValueUnits=m/s
  Pulley : Subsystem
      mask Display: image('pulley.png');
  Revolute Pulley : sm_lib/Joints/Revolute Joint  JointMode=Normal  SenseConstraintForce=off  SenseConstraintForceX=off  SenseConstraintForceY=off  SenseConstraintForceZ=off  SenseConstraintTorque=off  SenseConstraintTorqueX=off  SenseConstraintTorqueY=off  SenseConstraintTorqueZ=off  SenseTotalForce=off  SenseTotalForceX=off  SenseTotalForceY=off  SenseTotalForceZ=off  SenseTotalTorque=off  SenseTotalTorqueX=off  SenseTotalTorqueY=off  SenseTotalTorqueZ=off  CompositeWrenchDir=FollowerOnBase  CompositeWrenchFrame=BaseFrame  EquilibriumPosition=0  EquilibriumPositionUnits=deg  SpringStiffness=0  SpringStiffnessUnits=N*m/deg  DampingCoefficient=pulleyDamping  DampingCoefficientUnits=N*m/(deg/s)  TorqueActuationMode=NoTorque  MotionActuationMode=ComputedMotion  SensePosition=off  SenseVelocity=off  SenseAcceleration=off  SenseTorqueForce=off  SenseLowerLimitTorqueForce=off  SenseUpperLimitTorqueForce=off  LowerLimitSpecify=off  LowerLimitBound=-90  LowerLimitBoundUnits=deg  LowerLimitStiffness=1e4  LowerLimitStiffnessUnits=N*m/deg  LowerLimitDamping=10  LowerLimitDampingUnits=N*m/(deg/s)  LowerLimitTransitionRegionWidth=0.1  LowerLimitTransitionRegionWidthUnits=deg  UpperLimitSpecify=off  UpperLimitBound=90  UpperLimitBoundUnits=deg  UpperLimitStiffness=1e4  UpperLimitStiffnessUnits=N*m/deg  UpperLimitDamping=10  UpperLimitDampingUnits=N*m/(deg/s)  UpperLimitTransitionRegionWidth=0.1  UpperLimitTransitionRegionWidthUnits=deg  PositionTargetSpecify=off  PositionTargetPriority=High  PositionTargetValue=0  PositionTargetValueUnits=deg  VelocityTargetSpecify=off  VelocityTargetPriority=High  VelocityTargetValue=0  VelocityTargetValueUnits=deg/s
  Transform Cable End : sm_lib/Frames and Transforms/Rigid Transform  TranslationMethod=StandardAxis  TranslationStandardOffset=0.225+0.0075  TranslationLengthUnit=m  TranslationStandardAxis=+Y  TranslationCartesianOffset=[0 0 0]  TranslationROffset=0  TranslationROffsetUnits=m  TranslationZOffset=0  TranslationZOffsetUnits=m  TranslationThetaOffset=0  TranslationThetaOffsetUnits=deg  RotationMethod=None  RotationAngleUnits=deg  RotationStandardAxis=+Z  RotationAngle=0.0  RotationArbitraryAxis=[0 0 1]  FollAlignAxisA=+X  BaseAlignAxisA=+Y  FollAlignAxisB=+Y  BaseAlignAxisB=+Z  RotationSequenceAxes=FollowerAxes  RotationSequence=XYX  RotationSequenceAngles=[0 0 0]  RotationSequenceAnglesUnits=deg  RotationMatrix=[1 0 0; 0 1 0; 0 0 1]
  Transform Mass Constraint : sm_lib/Frames and Transforms/Rigid Transform  TranslationMethod=Cartesian  TranslationStandardOffset=0  TranslationLengthUnit=m  TranslationStandardAxis=+Z  TranslationCartesianOffset=[0 0 0]  TranslationROffset=0  TranslationROffsetUnits=m  TranslationZOffset=0  TranslationZOffsetUnits=m  TranslationThetaOffset=0  TranslationThetaOffsetUnits=deg  RotationMethod=StandardAxis  RotationAngleUnits=deg  RotationStandardAxis=+X  RotationAngle=-90  RotationArbitraryAxis=[0 0 1]  FollAlignAxisA=+X  BaseAlignAxisA=+Y  FollAlignAxisB=+Y  BaseAlignAxisB=+Z  RotationSequenceAxes=FollowerAxes  RotationSequence=XYX  RotationSequenceAngles=[0 0 0]  RotationSequenceAnglesUnits=deg  RotationMatrix=[1 0 0; 0 1 0; 0 0 1]
  Transform Prismatic : sm_lib/Frames and Transforms/Rigid Transform  TranslationMethod=Cartesian  TranslationStandardOffset=0  TranslationLengthUnit=m  TranslationStandardAxis=+Z  TranslationCartesianOffset="-[1.0560   -0.0300+1.1 0]"  TranslationROffset=0  TranslationROffsetUnits=m  TranslationZOffset=0  TranslationZOffsetUnits=m  TranslationThetaOffset=0  TranslationThetaOffsetUnits=deg  RotationMethod=StandardAxis  RotationAngleUnits=deg  RotationStandardAxis=+X  RotationAngle=-90  RotationArbitraryAxis=[0 0 1]  FollAlignAxisA=+X  BaseAlignAxisA=+Y  FollAlignAxisB=+Y  BaseAlignAxisB=+Z  RotationSequenceAxes=FollowerAxes  RotationSequence=XYX  RotationSequenceAngles=[0 0 0]  RotationSequenceAnglesUnits=deg  RotationMatrix=[1 0 0; 0 1 0; 0 0 1]
  Transform Pulley : sm_lib/Frames and Transforms/Rigid Transform  TranslationMethod=Cartesian  TranslationStandardOffset=0  TranslationLengthUnit=m  TranslationStandardAxis=+Z  TranslationCartesianOffset="[1.032  -0.209  0]"  TranslationROffset=0  TranslationROffsetUnits=m  TranslationZOffset=0  TranslationZOffsetUnits=m  TranslationThetaOffset=0  TranslationThetaOffsetUnits=deg  RotationMethod=None  RotationAngleUnits=deg  RotationStandardAxis=+Z  RotationAngle=0.0  RotationArbitraryAxis=[0 0 1]  FollAlignAxisA=+X  BaseAlignAxisA=+Y  FollAlignAxisB=+Y  BaseAlignAxisB=+Z  RotationSequenceAxes=FollowerAxes  RotationSequence=XYX  RotationSequenceAngles=[0 0 0]  RotationSequenceAnglesUnits=deg  RotationMatrix=[1 0 0; 0 1 0; 0 0 1]
  Cable : PMIOPort  Side=Left
  Bracket : PMIOPort  Port=2  Side=Left
  connections:
  Pulley/RConn1 -- Belt-Cable Properties/LConn1 -- Cable End Slider/RConn1
  Bracket/RConn1 -- Transform Prismatic/LConn1 -- Transform Pulley/RConn1
  Cable End Slider/LConn1 -- Transform Cable End/RConn1
  Transform Cable End/LConn1 -- Cable/RConn1
  Pulley/RConn2 -- Cable End Hook/RConn1
  Transform Pulley/LConn1 -- Revolute Pulley/LConn1
  Revolute Pulley/RConn1 -- Pulley/LConn1
  Hook/RConn1 -- Mass/RConn1 -- Transform Mass Constraint/LConn1
  Transform Prismatic/RConn1 -- Prismatic Hanging Mass/LConn1
  Prismatic Hanging Mass/RConn1 -- Transform Mass Constraint/RConn1
  Cable End Hook/LConn1 -- Hook/LConn1

== system airTrackLab/Air track model/Load/None ==
  Pulley : sm_lib/Body Elements/File Solid  ExtGeomFileName=wheel.stl  UnitType=Custom  ExtGeomFileUnits=mm  StepReaderType=HEX  ExportConvexHullGeometry=off  InertiaType=CalculateFromGeometry  Mass=180  MassUnits=g  CenterOfMass=[0 0 0]  CenterOfMassUnits=m  MomentsOfInertia=[1 1 1]  MomentsOfInertiaUnits=kg*m^2  ProductsOfInertia=[0 0 0]  ProductsOfInertiaUnits=kg*m^2  BasedOnType=Density  Density=1000  DensityUnits=kg/m^3  DoExposeReferenceFrame=off  SerializedFrames=<Frames><Frame><Id>Frame1</Id><Value><Name>F1</Name><Origin><Source>CenterOfMassFrame</Source><FeatureName></FeatureName></Origin><PrimaryAxis><DefinedDirection>+Z</DefinedDirection><Source>ReferenceFrame</Source><SourceDirection>+Z</SourceDirection><FeatureName></FeatureName></PrimaryAxis><SecondaryAxis><DefinedDirection>+Y</DefinedDirection><Source>ReferenceFrame</Source><SourceDirection>+Y</SourceDirection><FeatureName></FeatureName></SecondaryAxis></Value></Frame></Frames>  GraphicType=FromGeometry  MarkerShape=Sphere  MarkerSize=10  GraphicVisPropType=AdvancedVisualProperties  GraphicDiffuseColor="[0.8   0.8    0.8]"  GraphicSpecularColor="[0.8    0.8   0.8 1]"  GraphicAmbientColor=[0.05 0.05 0.05 1]  GraphicEmissiveColor=[0.0 0.0 0.0 1.0]  GraphicShininess=5  GraphicOpacity=1.0
  Reference Frame : sm_lib/Frames and Transforms/Reference Frame
  Transform Pulley : sm_lib/Frames and Transforms/Rigid Transform  TranslationMethod=Cartesian  TranslationStandardOffset=0  TranslationLengthUnit=m  TranslationStandardAxis=+Z  TranslationCartesianOffset="[1.032  -0.209  0]"  TranslationROffset=0  TranslationROffsetUnits=m  TranslationZOffset=0  TranslationZOffsetUnits=m  TranslationThetaOffset=0  TranslationThetaOffsetUnits=deg  RotationMethod=None  RotationAngleUnits=deg  RotationStandardAxis=+Z  RotationAngle=0.0  RotationArbitraryAxis=[0 0 1]  FollAlignAxisA=+X  BaseAlignAxisA=+Y  FollAlignAxisB=+Y  BaseAlignAxisB=+Z  RotationSequenceAxes=FollowerAxes  RotationSequence=XYX  RotationSequenceAngles=[0 0 0]  RotationSequenceAnglesUnits=deg  RotationMatrix=[1 0 0; 0 1 0; 0 0 1]
  Cable : PMIOPort  Side=Left
  Bracket : PMIOPort  Port=2  Side=Left
  connections:
  Cable/RConn1 -- Reference Frame/RConn1
  Transform Pulley/RConn1 -- Bracket/RConn1
  Transform Pulley/LConn1 -- Pulley/LConn1

== system airTrackLab/Air track model/Mass Cart 1/None  ==
  Reference Frame : sm_lib/Frames and Transforms/Reference Frame
  B : PMIOPort  Side=Right
  connections:
  B/RConn1 -- Reference Frame/RConn1

== system airTrackLab/Air track model/Mass Cart 1/Plates 1 ==
  Plate 1 : sm_lib/Body Elements/File Solid  ExtGeomFileName=weight.stl  UnitType=Custom  ExtGeomFileUnits=mm  StepReaderType=HEX  ExportConvexHullGeometry=off  InertiaType=PointMass  Mass=100  MassUnits=g  CenterOfMass=[0 0 0]  CenterOfMassUnits=m  MomentsOfInertia=[1 1 1]  MomentsOfInertiaUnits=kg*m^2  ProductsOfInertia=[0 0 0]  ProductsOfInertiaUnits=kg*m^2  BasedOnType=Density  Density=1000  DensityUnits=kg/m^3  DoExposeReferenceFrame=on  SerializedFrames=<Frames/>  GraphicType=FromGeometry  MarkerShape=Sphere  MarkerSize=10  GraphicVisPropType=AdvancedVisualProperties  GraphicDiffuseColor="[0.70   0.7    0.3]"  GraphicSpecularColor="[0.7  0.7  0.5 1]"  GraphicAmbientColor=[0.05 0.05 0.05 1]  GraphicEmissiveColor=[0.2 0.2 0.2 1.0]  GraphicShininess=3  GraphicOpacity=1.0
  Transform Plate 1 : sm_lib/Frames and Transforms/Rigid Transform  TranslationMethod=Cartesian  TranslationStandardOffset=0  TranslationLengthUnit=m  TranslationStandardAxis=+Z  TranslationCartesianOffset=[0 0.0055 0.0]  TranslationROffset=0  TranslationROffsetUnits=m  TranslationZOffset=0  TranslationZOffsetUnits=m  TranslationThetaOffset=0  TranslationThetaOffsetUnits=deg  RotationMethod=None  RotationAngleUnits=deg  RotationStandardAxis=+Z  RotationAngle=0.0  RotationArbitraryAxis=[0 0 1]  FollAlignAxisA=+X  BaseAlignAxisA=+Y  FollAlignAxisB=+Y  BaseAlignAxisB=+Z  RotationSequenceAxes=FollowerAxes  RotationSequence=XYX  RotationSequenceAngles=[0 0 0]  RotationSequenceAnglesUnits=deg  RotationMatrix=[1 0 0; 0 1 0; 0 0 1]
  B : PMIOPort  Side=Right
  connections:
  Transform Plate 1/LConn1 -- B/RConn1
  Plate 1/RConn1 -- Transform Plate 1/RConn1

== system airTrackLab/Air track model/Mass Cart 1/Plates 2 ==
  Plate 1 : sm_lib/Body Elements/File Solid  ExtGeomFileName=weight.stl  UnitType=Custom  ExtGeomFileUnits=mm  StepReaderType=HEX  ExportConvexHullGeometry=off  InertiaType=PointMass  Mass=100  MassUnits=g  CenterOfMass=[0 0 0]  CenterOfMassUnits=m  MomentsOfInertia=[1 1 1]  MomentsOfInertiaUnits=kg*m^2  ProductsOfInertia=[0 0 0]  ProductsOfInertiaUnits=kg*m^2  BasedOnType=Density  Density=1000  DensityUnits=kg/m^3  DoExposeReferenceFrame=on  SerializedFrames=<Frames/>  GraphicType=FromGeometry  MarkerShape=Sphere  MarkerSize=10  GraphicVisPropType=AdvancedVisualProperties  GraphicDiffuseColor="[0.70   0.7    0.3]"  GraphicSpecularColor="[0.7  0.7  0.5 1]"  GraphicAmbientColor=[0.05 0.05 0.05 1]  GraphicEmissiveColor=[0.2 0.2 0.2 1.0]  GraphicShininess=3  GraphicOpacity=1.0
  Plate 2 : sm_lib/Body Elements/File Solid  ExtGeomFileName=weight.stl  UnitType=Custom  ExtGeomFileUnits=mm  StepReaderType=HEX  ExportConvexHullGeometry=off  InertiaType=PointMass  Mass=100  MassUnits=g  CenterOfMass=[0 0 0]  CenterOfMassUnits=m  MomentsOfInertia=[1 1 1]  MomentsOfInertiaUnits=kg*m^2  ProductsOfInertia=[0 0 0]  ProductsOfInertiaUnits=kg*m^2  BasedOnType=Density  Density=1000  DensityUnits=kg/m^3  DoExposeReferenceFrame=on  SerializedFrames=<Frames/>  GraphicType=FromGeometry  MarkerShape=Sphere  MarkerSize=10  GraphicVisPropType=AdvancedVisualProperties  GraphicDiffuseColor="[0.70   0.7    0.3]"  GraphicSpecularColor="[0.7  0.7  0.5 1]"  GraphicAmbientColor=[0.05 0.05 0.05 1]  GraphicEmissiveColor=[0.2 0.2 0.2 1.0]  GraphicShininess=3  GraphicOpacity=1.0
  Transform Plate 1 : sm_lib/Frames and Transforms/Rigid Transform  TranslationMethod=Cartesian  TranslationStandardOffset=0  TranslationLengthUnit=m  TranslationStandardAxis=+Z  TranslationCartesianOffset=[0 0.0055 0.0]  TranslationROffset=0  TranslationROffsetUnits=m  TranslationZOffset=0  TranslationZOffsetUnits=m  TranslationThetaOffset=0  TranslationThetaOffsetUnits=deg  RotationMethod=None  RotationAngleUnits=deg  RotationStandardAxis=+Z  RotationAngle=0.0  RotationArbitraryAxis=[0 0 1]  FollAlignAxisA=+X  BaseAlignAxisA=+Y  FollAlignAxisB=+Y  BaseAlignAxisB=+Z  RotationSequenceAxes=FollowerAxes  RotationSequence=XYX  RotationSequenceAngles=[0 0 0]  RotationSequenceAnglesUnits=deg  RotationMatrix=[1 0 0; 0 1 0; 0 0 1]
  Transform Plate 2 : sm_lib/Frames and Transforms/Rigid Transform  TranslationMethod=Cartesian  TranslationStandardOffset=0  TranslationLengthUnit=m  TranslationStandardAxis=+Z  TranslationCartesianOffset=[0 0.0055 0.0]  TranslationROffset=0  TranslationROffsetUnits=m  TranslationZOffset=0  TranslationZOffsetUnits=m  TranslationThetaOffset=0  TranslationThetaOffsetUnits=deg  RotationMethod=None  RotationAngleUnits=deg  RotationStandardAxis=+Z  RotationAngle=0.0  RotationArbitraryAxis=[0 0 1]  FollAlignAxisA=+X  BaseAlignAxisA=+Y  FollAlignAxisB=+Y  BaseAlignAxisB=+Z  RotationSequenceAxes=FollowerAxes  RotationSequence=XYX  RotationSequenceAngles=[0 0 0]  RotationSequenceAnglesUnits=deg  RotationMatrix=[1 0 0; 0 1 0; 0 0 1]
  B : PMIOPort  Side=Right
  connections:
  Plate 1/RConn1 -- Transform Plate 2/LConn1 -- Transform Plate 1/RConn1
  Transform Plate 1/LConn1 -- B/RConn1
  Plate 2/RConn1 -- Transform Plate 2/RConn1
